simulink model "A5_model_controller"  (R2025b)
settings: Solver=VariableStepAuto  StartTime=0.0  StopTime=timeSim  FixedStep=0.00001  MaxStep=1e-3  RelTol=1e-3
undefined symbols (not defined in the file): Bf, Bk, Br, Cf, Ck, Ckappa, Cr, Cyf, Cyr, Df, Dk, Dr, eps_num, h, Izz, Jw, K_aug, K_T, Kr_T, lf, lr, m, Rw, tr, vx
libraries: simulink_extras x3, cstblocks x1
settings Model: Creator=jofr  LastModifiedBy=danilo
settings SolverCC: AlgebraicLoopSolver=TrustRegion
settings DataIOCC: LimitDataPoints=on  SaveFormat=Array  SignalLoggingSaveFormat=ModelDataLogs  ReturnWorkspaceOutputs=off
settings OptimizationCC: BlockReduction=off  BooleanDataType=off  DefaultParameterBehavior=Inlined  BufferReuse=off  LifeSpan=inf
settings DebuggingCC: SaveWithParameterizedLinksMsg=none  UnderspecifiedInitializationDetection=Classic  MergeDetectMultiDrivingBlocksExec=none  SignalResolutionControl=TryResolveAllWithWarning  MultiTaskDSMMsg=warning  MultiTaskCondExecSysMsg=none  UnconnectedInputMsg=warning  UnconnectedOutputMsg=warning  UnconnectedLineMsg=warning  InitInArrayFormatMsg=none  SFUnexpectedBacktrackingDiag=warning  SFNoUnconditionalDefaultTransitionDiag=warning  SFExecutionAtInitializationDiag=none  ArithmeticOperatorsInVariantConditions=warning
settings HardwareCC: ProdBitPerPointer=32.0  ProdBitPerSizeT=32.0  ProdBitPerPtrDiffT=32.0  ProdLargestAtomicFloat=None  ProdIntDivRoundTo=Undefined  ProdEndianess=Unspecified  ProdWordSize=32.0  ProdHWDeviceType=32-bit Generic  TargetUnknown=on
settings ModelReferenceCC: EnableRefExpFcnMdlSchedulingChecks=on  PropagateSignalLabelsOutOfModel=off
settings SFSimCC: SimUseLocalCustomCode=off  CustomCodeUndefinedFunction=UseInterfaceOnly
settings RTWCC: RTWUseLocalCustomCode=off  GPUComputeCapability=3.5  DLArmComputeVersion=19.05
settings CodeAppCC: StateflowObjectComments=on
settings GRTTargetCC: TargetLangStandard=C89/C90 (ANSI)
settings ConfigComp: CovMetricSettings=dw  CovSaveCumulativeToWorkspaceVar=on  CovSaveSingleToWorkspaceVar=on  CovExternalEMLEnable=off

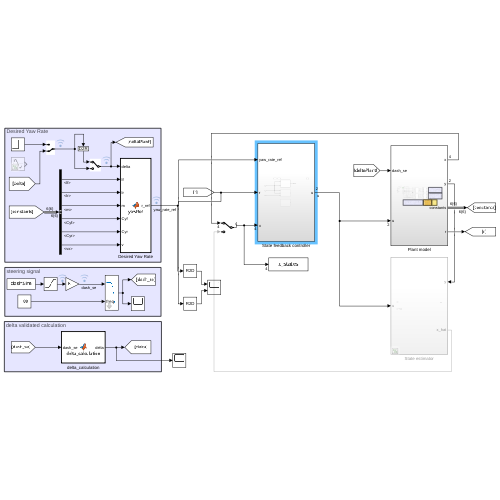
[thumbnail: Simulink's stored preview of the top-level diagram]
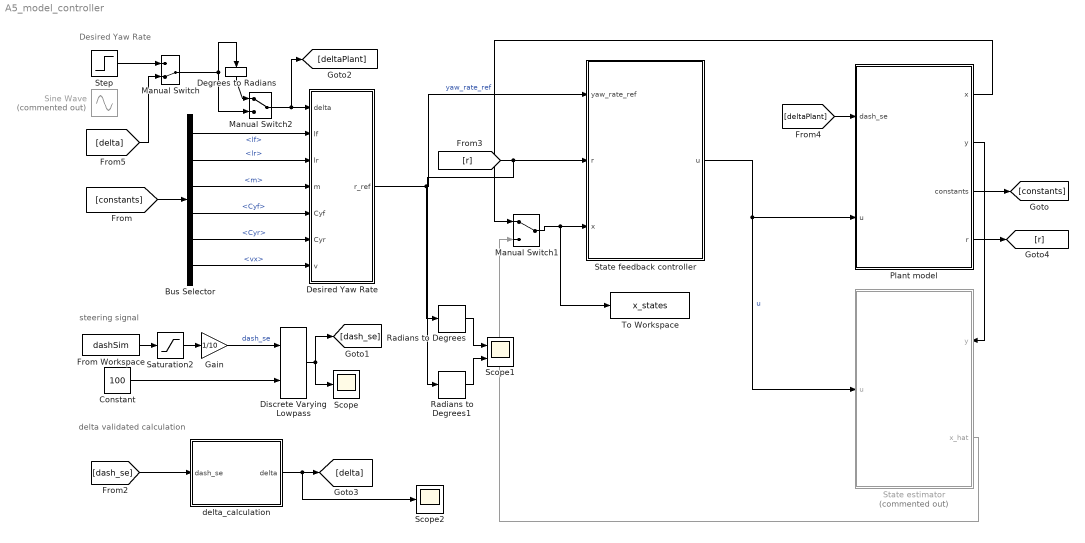
== system A5_model_controller ==
  note: delta validated calculation
  note: steering signal
  note: Desired Yaw Rate
  Bus Selector : BusSelector  OutputSignals=lf,lr,m,Cyf,Cyr,vx
  Constant : Constant  Value=100
  Degrees to Radians : simulink_extras/Transformations/Degrees to Radians
  Desired Yaw Rate : MATLAB Function  TreatAsAtomicUnit=on
  Discrete Varying Lowpass : cstblocks/Linear Parameter Varying/Discrete Varying Lowpass  N=1  w0=0  Ts=0.01
  From Workspace : FromWorkspace  VariableName=dashSim
  Gain : Gain  Gain=1/10
  Manual Switch : ManualSwitch  CurrentSetting=0
  Manual Switch1 : ManualSwitch
  Manual Switch2 : ManualSwitch
  Plant model : Subsystem
  Radians to Degrees : simulink_extras/Transformations/Radians to Degrees
  Radians to Degrees1 : simulink_extras/Transformations/Radians to Degrees
  Saturation2 : Saturate  UpperLimit=1270  LowerLimit=-1270
  Scope : Scope
      settings: ActiveDisplayYMinimum=-354.89564145632545  ActiveDisplayYMaximum=435.3727455414014  DataLoggingVariableName=ScopeData13
  Scope1 : Scope  NumInputPorts=2
      settings: ActiveDisplayYMinimum=-206.00372470004959  ActiveDisplayYMaximum=1854.0335223004467  DataLoggingVariableName=ScopeData12
  Scope2 : Scope
      settings: ActiveDisplayYMinimum=-1  ActiveDisplayYMaximum=1  DataLoggingVariableName=ScopeData18
  Sine Wave : Sin  Commented=on  Amplitude=10*(pi()/180)  Frequency=5  SampleTime=0
  State estimator : Subsystem  Commented=on
      settings: PortSchema="{\"entries\":[{\"content\":{\"sides\":[{\"content\":{\"connectorIds\":[\"In1\"]},\"type\":\"ConnectorPlacement.EquallySpacedRectSide\",\"uuid\":\"c417f3d4-912d-40bf-9a3a-53ea69fe223c\"},{\"content\":{\"connectorIds\":[\"In2\",\"Out1\"],\"side\":\"RIGHT\"},\"type\":\"ConnectorPlacement.EquallySpacedRectSide\",\"uuid\":\"4e25e672-d4ae-48e6-baf9-37985f0fdcbd\"},{\"content\":{\"connectorIds\":[],\"side\":\"TOP\"},\"type\":\"ConnectorPlacement.EquallySpacedRectSide\",\"uuid\":\"19dfc206-a33d-4b15-9300-bad270a3e9d6\"},{\"content\":{\"connectorIds\":[],\"side\":\"HIDDEN\"},\"type\":\"ConnectorPlacement.EquallySpacedRectSide\",\"uuid\":\"ab455fac-7bff-4c9f-9be5-2f044e5e011f\"}]},\"type\":\"ConnectorPlacement.EquallySpacedConnector\",\"uuid\":\"aea33454-8eab-4b9c-b4de-a2355e2c58aa\"}],\"packageUris\":[\"http://schema.mathworks.com/mf0/Connector/R2020b\"],\"version\":\"1.0\"}"
  State feedback controller : Subsystem
  Step : Step  SampleTime=0
  To Workspace : ToWorkspace  VariableName=x_states  SaveFormat=Structure With Time  SampleTime=-1
  delta_calculation : MATLAB Function  TreatAsAtomicUnit=on
  wires:
  State feedback controller/1(u) -> State estimator/1(u), Plant model/2(u)  "u"
  Plant model/2(y) -> State estimator/2(y)
  Manual Switch1/1 -> To Workspace/1, State feedback controller/3(x)
  State estimator/1(x_hat) -> Manual Switch1/2
  Plant model/1(x) -> Manual Switch1/1
  Plant model/3(constants) -> [constants]
  [constants] -> Bus Selector/1
  Bus Selector/1 -> Desired Yaw Rate/2(lf)  "<lf>"
  Bus Selector/2 -> Desired Yaw Rate/3(lr)  "<lr>"
  Bus Selector/3 -> Desired Yaw Rate/4(m)  "<m>"
  Bus Selector/4 -> Desired Yaw Rate/5(Cyf)  "<Cyf>"
  Bus Selector/5 -> Desired Yaw Rate/6(Cyr)  "<Cyr>"
  Bus Selector/6 -> Desired Yaw Rate/7(v)  "<vx>"
  From Workspace/1 -> Saturation2/1
  Saturation2/1 -> Gain/1
  Gain/1 -> Discrete Varying Lowpass/1  "dash_se"
  Discrete Varying Lowpass/1 -> [dash_se], Scope/1
  Constant/1 -> Discrete Varying Lowpass/2
  Manual Switch/1 -> Manual Switch2/2, Degrees to Radians/1
  Degrees to Radians/1 -> Manual Switch2/1
  Manual Switch2/1 -> [deltaPlant], Desired Yaw Rate/1(delta)
  Step/1 -> Manual Switch/1
  Desired Yaw Rate/1(r_ref) -> Radians to Degrees/1, State feedback controller/1(yaw_rate_ref)  "yaw_rate_ref"
  [dash_se] -> delta_calculation/1(dash_se)
  delta_calculation/1(delta) -> Scope2/1, [delta]
  Plant model/4(r) -> [r]
  [r] -> Radians to Degrees1/1, State feedback controller/2(r)
  Radians to Degrees/1 -> Scope1/1
  Radians to Degrees1/1 -> Scope1/2
  [deltaPlant] -> Plant model/1(dash_se)
  [delta] -> Manual Switch/2

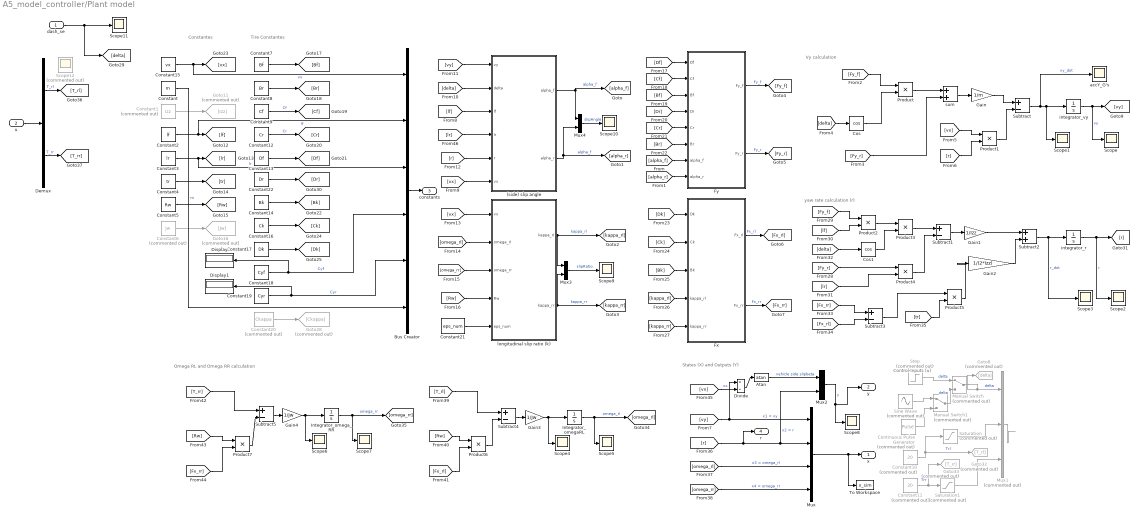
== system A5_model_controller/Plant model ==
  note: Constantes
  note: Omega RL and Omega RR calculation
  note: Control Inputs (u)
  note: States (X) and Outputs (Y)
  note: yaw rate calculation (r)
  note: Vy calculation
  note: Tire Constantes
  dash_se : Inport
  u : Inport  Port=2  PortDimensions=2
  (side) slip angle : MATLAB Function  TreatAsAtomicUnit=on
  Atan : Trigonometry  Operator=atan
  Bus Creator : BusCreator  Inputs=6
  Constant : Constant  Value=m
  Constant1 : Constant  Commented=on  Value=Izz
  Constant10 : Constant  Commented=on  Value=20
  Constant11 : Constant  Commented=on  Value=20
  Constant12 : Constant  Value=Cr
  Constant13 : Constant  Value=Df
  Constant14 : Constant  Value=Bk
  Constant15 : Constant  Value=vx
  Constant16 : Constant  Value=Ck
  Constant17 : Constant  Value=Dk
  Constant18 : Constant  Value=Cyf
  Constant19 : Constant  Value=Cyr
  Constant2 : Constant  Value=lf
  Constant20 : Constant  Commented=on  Value=Ckappa
  Constant21 : Constant  Value=eps_num
  Constant22 : Constant  Value=Dr
  Constant3 : Constant  Value=lr
  Constant4 : Constant  Value=tr
  Constant5 : Constant  Value=Rw
  Constant6 : Constant  Commented=on  Value=Jw
  Constant7 : Constant  Value=Bf
  Constant8 : Constant  Value=Br
  Constant9 : Constant  Value=Cf
  Continuous Pulse Generator : DiscretePulseGenerator  Commented=on  PulseType=Time based  Period=1  PulseWidth=50
  Cos : Trigonometry  Operator=cos
  Cos1 : Trigonometry  Operator=cos
  Demux : Demux  Outputs=2
  Display : Display
  Display1 : Display
  Divide : Product  Inputs=*/
  Fx : MATLAB Function  TreatAsAtomicUnit=on
  Fy : MATLAB Function  TreatAsAtomicUnit=on
  Gain : Gain  Gain=1/m
  Gain1 : Gain  Gain=1/Izz
  Gain2 : Gain  Gain=1/(2*Izz)
  Gain3 : Gain  Gain=1/Jw
  Gain4 : Gain  Gain=1/Jw
  Goto11 : Goto  Commented=on  GotoTag=Izz
  Goto16 : Goto  Commented=on  GotoTag=Jw
  Goto28 : Goto  Commented=on  GotoTag=Ckappa
  Goto32 : Goto  Commented=on  GotoTag=T_rl
  Goto33 : Goto  Commented=on  GotoTag=T_rr
  Goto8 : Goto  Commented=on  GotoTag=delta
  Integrator_omegaRL : Integrator  InitialCondition=vx/Rw
  Integrator_omega_RR : Integrator  InitialCondition=vx/Rw
  Manual Switch : ManualSwitch  Commented=on
  Manual Switch1 : ManualSwitch  Commented=on
  Mux : Mux
  Mux1 : Mux  Commented=on  Inputs=3
  Mux2 : Mux  Inputs=2
  Mux3 : Mux  Inputs=2
  Mux4 : Mux  Inputs=2
  Product{,1..7} (8 alike) : Product
  Saturation : Saturate  Commented=on
  Saturation1 : Saturate  Commented=on
  Scope{,1..11} (12 alike) : Scope
      Scope settings: ActiveDisplayYMinimum=-1  ActiveDisplayYMaximum=1
      Scope10 settings: ActiveDisplayYMinimum=-1  ActiveDisplayYMaximum=1  DataLoggingVariableName=ScopeData10
      Scope11 settings: DataLoggingVariableName=ScopeData14
      Scope2 settings: ActiveDisplayYMinimum=-11.738874514113046  ActiveDisplayYMaximum=1.5902174171245722  DataLoggingVariableName=ScopeData2
      Scope3 settings: DataLoggingVariableName=ScopeData3
      Scope4 settings: ActiveDisplayYMinimum=-1  ActiveDisplayYMaximum=1  DataLoggingVariableName=ScopeData4
      Scope5 settings: ActiveDisplayYMinimum=-1  ActiveDisplayYMaximum=1  DataLoggingVariableName=ScopeData5
      Scope6 settings: ActiveDisplayYMinimum=-1  ActiveDisplayYMaximum=1  DataLoggingVariableName=ScopeData6
      Scope7 settings: ActiveDisplayYMinimum=-1  ActiveDisplayYMaximum=1  DataLoggingVariableName=ScopeData7
      Scope8 settings: ActiveDisplayYMinimum=-1  ActiveDisplayYMaximum=1  DataLoggingVariableName=ScopeData8
      Scope9 settings: ActiveDisplayYMinimum=-1  ActiveDisplayYMaximum=1  DataLoggingVariableName=ScopeData9
  Scope12 : Scope  Commented=on
      settings: ActiveDisplayYMinimum=-0.01610091878561485  ActiveDisplayYMaximum=0.0017936004292760203  DataLoggingVariableName=ScopeData15
  Sine Wave : Sin  Commented=on  SampleTime=0
  Step : Step  Commented=on  SampleTime=0
  Subtract{,1,3..5} (5 alike) : Sum  Inputs=+-
  Subtract2 : Sum
  To Workspace : ToWorkspace  VariableName=x_sim  SaveFormat=Structure With Time  SampleTime=-1
  accY_G's : Scope
      settings: DataLoggingVariableName=ScopeData11
  integrator_r : Integrator
  integrator_vy : Integrator
  "longitudinal slip ratio (k) " : MATLAB Function  TreatAsAtomicUnit=on
  sum : Sum
  x : Outport
  y : Outport  Port=2
  constants : Outport  Port=3
  r : Outport  Port=4
  wires:
  [vy] -> Divide/1, Mux/1  "x1 = vy"
  [r] -> r/1, Mux/2, Mux2/2  "x2 = r"
  Constant10/1 -> Saturation/1, Goto32/1  "Trl"
  Constant11/1 -> Goto33/1, Saturation1/1  "Trr"
  (side) slip angle/1(alpha_f) -> [alpha_f], Mux4/1  "alpha_f"
  (side) slip angle/2(alpha_r) -> Mux4/2, [alpha_r]  "alpha_f"
  "longitudinal slip ratio (k) "/1(kappa_rl) -> [kappa_rl], Mux3/1  "kappa_rl"
  "longitudinal slip ratio (k) "/2(kappa_rr) -> [kappa_rr], Mux3/2  "kappa_rr"
  Fy/1(Fy_f) -> [Fy_f]  "Fy_f"
  Fy/2(Fy_r) -> [Fy_r]  "Fy_r"
  Fx/1(Fx_rl) -> [Fx_rl]  "Fx_rl"
  Fx/2(Fx_rr) -> [Fx_rr]  "Fx_rr"
  [alpha_f] -> Fy/7(alpha_f)
  [alpha_r] -> Fy/8(alpha_r)
  [delta] -> Cos/1
  [Fy_f] -> Product/1
  Cos/1 -> Product/2
  Product/1 -> sum/1
  [Fy_r] -> sum/2
  sum/1 -> Gain/1
  Gain/1 -> Subtract/1
  [vx] -> Product1/1
  [r] -> Product1/2
  Product1/1 -> Subtract/2
  Subtract/1 -> accY_G's/1, Scope1/1, integrator_vy/1  "vy_dot"
  integrator_vy/1 -> Scope/1, [vy]  "vy"
  Constant1/1 -> Goto11/1
  Constant2/1 -> [lf], Bus Creator/2  "lf"
  Constant3/1 -> [lr], Bus Creator/3  "lr"
  Constant4/1 -> [tr]
  Constant5/1 -> [Rw]
  Constant6/1 -> Goto16/1
  Constant7/1 -> [Bf]
  Constant8/1 -> [Br]
  Constant9/1 -> [Cf]  "Cf"
  Constant12/1 -> [Cr]  "Cr"
  Constant13/1 -> [Df]
  Constant14/1 -> [Bk]
  Constant15/1 -> Bus Creator/1, [vx]  "vx"
  Constant16/1 -> [Ck]
  Constant17/1 -> [Dk]
  Constant18/1 -> Display/1, Bus Creator/4  "Cyf"
  Constant19/1 -> Display1/1, Bus Creator/5  "Cyr"
  Constant20/1 -> Goto28/1
  [vx] -> (side) slip angle/6(vx)
  [vy] -> (side) slip angle/1(vy)
  [delta] -> (side) slip angle/2(delta)
  [lf] -> (side) slip angle/3(lf)
  [r] -> (side) slip angle/5(r)
  [vx] -> "longitudinal slip ratio (k) "/1(vx)
  [omega_rl] -> "longitudinal slip ratio (k) "/2(omega_rl)
  [Rw] -> "longitudinal slip ratio (k) "/4(Rw)
  [omega_rr] -> "longitudinal slip ratio (k) "/3(omega_rr)
  [Df] -> Fy/1(Df)
  [Cf] -> Fy/2(Cf)
  [Bf] -> Fy/3(Bf)
  [Dr] -> Fy/4(Dr)
  [Cr] -> Fy/5(Cr)
  [Br] -> Fy/6(Br)
  Constant22/1 -> [Dr]
  Saturation/1 -> Mux1/2
  Saturation1/1 -> Mux1/3
  [Dk] -> Fx/1(Dk)
  [Ck] -> Fx/2(Ck)
  [Bk] -> Fx/3(Bk)
  [kappa_rl] -> Fx/4(kappa_rl)
  [kappa_rr] -> Fx/5(kappa_rr)
  [delta] -> Cos1/1
  [Fy_f] -> Product2/1
  [lf] -> Product2/2
  Cos1/1 -> Product3/2
  Product2/1 -> Product3/1
  [Fy_r] -> Product4/1
  [lr] -> Product4/2
  Product4/1 -> Subtract1/2
  Product3/1 -> Subtract1/1
  Subtract1/1 -> Gain1/1
  [Fx_rr] -> Subtract3/1
  [Fx_rl] -> Subtract3/2
  Subtract3/1 -> Product5/1
  [tr] -> Product5/2
  Product5/1 -> Gain2/1
  Gain2/1 -> Subtract2/2
  Subtract2/1 -> Scope3/1, integrator_r/1  "r_dot"
  [Rw] -> Product6/1
  [Fx_rl] -> Product6/2
  Product6/1 -> Subtract4/2
  [T_rl] -> Subtract4/1
  Subtract4/1 -> Gain3/1
  Gain3/1 -> Scope4/1, Integrator_omegaRL/1
  Integrator_omegaRL/1 -> Scope5/1, [omega_rl]  "omega_rl"
  Integrator_omega_RR/1 -> [omega_rr], Scope7/1  "omega_rr"
  Gain4/1 -> Integrator_omega_RR/1, Scope6/1
  Subtract5/1 -> Gain4/1
  [T_rr] -> Subtract5/1
  Product7/1 -> Subtract5/2
  [Fx_rr] -> Product7/2
  [Rw] -> Product7/1
  Mux2/1 -> Scope8/1, y/1  "y"
  Atan/1 -> Mux2/1  "vehicle side slipbeta"
  Divide/1 -> Atan/1
  [vx] -> Divide/2  "vx"
  Constant/1 -> Bus Creator/6  "m"
  [lr] -> (side) slip angle/4(lr)
  Mux3/1 -> Scope9/1  "slipRatio"
  Mux4/1 -> Scope10/1  "slipAngle"
  Manual Switch/1 -> Goto8/1, Mux1/1  "delta"
  Step/1 -> Manual Switch/1  "delta"
  Continuous Pulse Generator/1 -> Manual Switch1/2
  Manual Switch1/1 -> Manual Switch/2  "delta"
  Sine Wave/1 -> Manual Switch1/1
  Mux1/1 -> ?
  u/1 -> Demux/1
  Constant21/1 -> "longitudinal slip ratio (k) "/5(eps_num)
  Bus Creator/1 -> constants/1
  Mux/1 -> To Workspace/1, x/1
  Gain1/1 -> Subtract2/1
  integrator_r/1 -> Scope2/1, [r]  "r"
  [omega_rl] -> Mux/3  "x3 = omega_rl"
  [omega_rr] -> Mux/4  "x4 = omega_rr"
  dash_se/1 -> [delta], Scope11/1
  Demux/1 -> [T_rl]  "T_rl"
  Demux/2 -> [T_rr]  "T_rr"

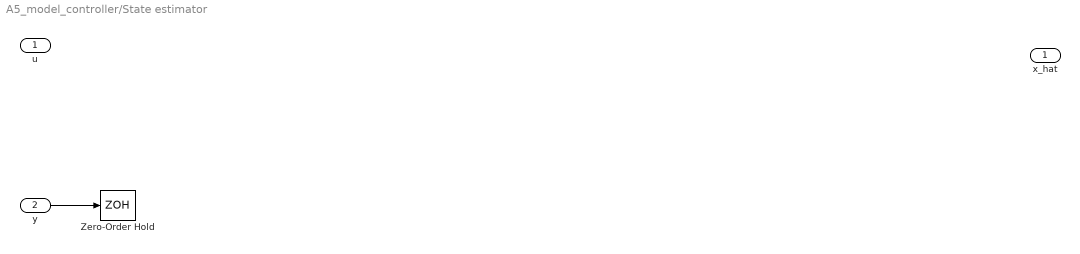
== system A5_model_controller/State estimator ==
  u : Inport
  y : Inport  Port=2
  Zero-Order Hold : ZeroOrderHold  SampleTime=h
  x_hat : Outport
  wires:
  y/1 -> Zero-Order Hold/1

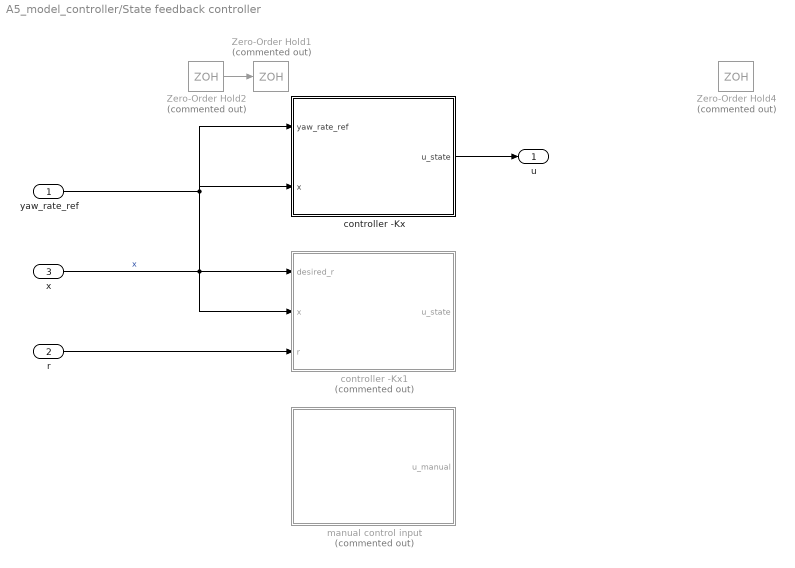
== system A5_model_controller/State feedback controller ==
  yaw_rate_ref : Inport
  r : Inport  Port=2
  x : Inport  Port=3
  Zero-Order Hold1 : ZeroOrderHold  Commented=on  SampleTime=h
  Zero-Order Hold2 : ZeroOrderHold  Commented=on  SampleTime=h
  Zero-Order Hold4 : ZeroOrderHold  Commented=on  SampleTime=-1
  controller -Kx : Subsystem
  controller -Kx1 : Subsystem  Commented=on
  manual control input : Subsystem  Commented=on
  u : Outport  PortDimensions=2
  wires:
  Zero-Order Hold2/1 -> Zero-Order Hold1/1
  yaw_rate_ref/1 -> controller -Kx1/1(desired_r), controller -Kx/1(yaw_rate_ref)
  x/1 -> controller -Kx/2(x), controller -Kx1/2(x)  "x"
  r/1 -> controller -Kx1/3(r)
  controller -Kx/1(u_state) -> u/1

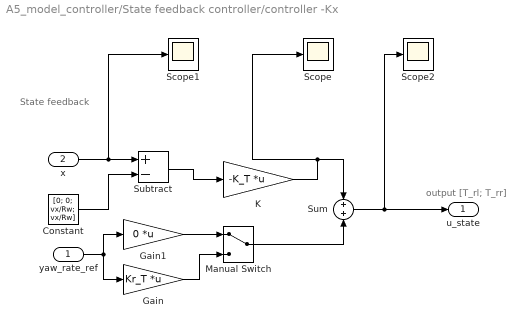
== system A5_model_controller/State feedback controller/controller -Kx ==
  note: output [T_rl; T_rr]
  note: State feedback
  yaw_rate_ref : Inport
  x : Inport  Port=2  PortDimensions=4
  Constant : Constant  Value=[0; 0; vx/Rw; vx/Rw]  VectorParams1D=off
  Gain : Gain  Gain=Kr_T  Multiplication=Matrix(K*u)
  Gain1 : Gain  Gain=0  Multiplication=Matrix(K*u)
  K : Gain  Gain=-K_T  Multiplication=Matrix(K*u)
  Manual Switch : ManualSwitch
  Scope : Scope
      settings: ActiveDisplayYMinimum=-0.0010140194157633876  ActiveDisplayYMaximum=0.0010146249929807261  DataLoggingVariableName=ScopeData16
  Scope1 : Scope
      settings: ActiveDisplayYMinimum=-6.7509721632618485  ActiveDisplayYMaximum=49.483096533791262  DataLoggingVariableName=ScopeData17
  Scope2 : Scope
      settings: ActiveDisplayYMinimum=-0.41126063504540261  ActiveDisplayYMaximum=0.41126063504546317  DataLoggingVariableName=ScopeData19
  Subtract : Sum  Inputs=+-
  Sum : Sum
  u_state : Outport  PortDimensions=2
  wires:
  x/1 -> Subtract/1, Scope1/1
  K/1 -> Scope/1, Sum/1
  Sum/1 -> Scope2/1, u_state/1
  Gain/1 -> Manual Switch/2
  yaw_rate_ref/1 -> Gain/1, Gain1/1
  Manual Switch/1 -> Sum/2
  Gain1/1 -> Manual Switch/1
  Subtract/1 -> K/1
  Constant/1 -> Subtract/2

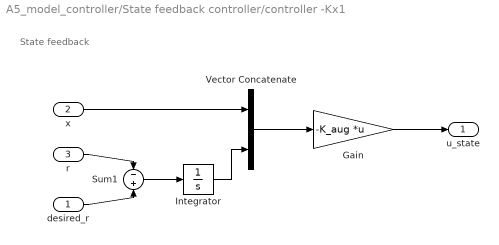
== system A5_model_controller/State feedback controller/controller -Kx1 ==
  note: State feedback
  desired_r : Inport
  x : Inport  Port=2  PortDimensions=4
  r : Inport  Port=3
  Gain : Gain  Gain=-K_aug  Multiplication=Matrix(K*u)
  Integrator : Integrator
  Sum1 : Sum  Inputs=-+
  Vector Concatenate : Concatenate
  u_state : Outport
  wires:
  desired_r/1 -> Sum1/2
  x/1 -> Vector Concatenate/1
  r/1 -> Sum1/1
  Sum1/1 -> Integrator/1
  Vector Concatenate/1 -> Gain/1
  Integrator/1 -> Vector Concatenate/2
  Gain/1 -> u_state/1

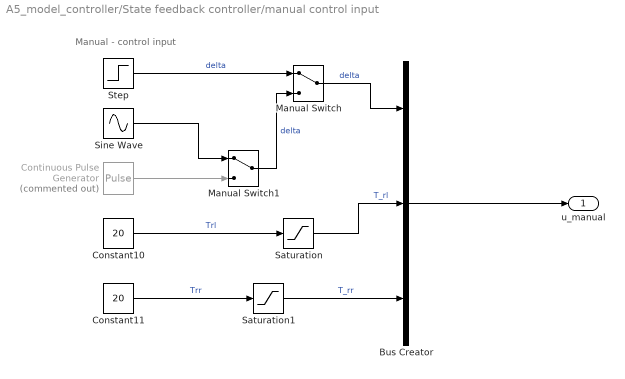
== system A5_model_controller/State feedback controller/manual control input ==
  note: Manual - control input
  Bus Creator : BusCreator  Inputs=3
  Constant10 : Constant  Value=20
  Constant11 : Constant  Value=20
  Continuous Pulse Generator : DiscretePulseGenerator  Commented=on  PulseType=Time based  Period=1  PulseWidth=50
  Manual Switch : ManualSwitch
  Manual Switch1 : ManualSwitch
  Saturation : Saturate
  Saturation1 : Saturate
  Sine Wave : Sin  SampleTime=0
  Step : Step  SampleTime=0
  u_manual : Outport
  wires:
  Sine Wave/1 -> Manual Switch1/1
  Manual Switch/1 -> Bus Creator/1  "delta"
  Constant11/1 -> Saturation1/1  "Trr"
  Continuous Pulse Generator/1 -> Manual Switch1/2
  Manual Switch1/1 -> Manual Switch/2  "delta"
  Saturation1/1 -> Bus Creator/3  "T_rr"
  Saturation/1 -> Bus Creator/2  "T_rl"
  Constant10/1 -> Saturation/1  "Trl"
  Bus Creator/1 -> u_manual/1
  Step/1 -> Manual Switch/1  "delta"

== matlab function A5_model_controller/Plant model/longitudinal slip ratio (k)  ==
  data: vx input; kappa_rl output; omega_rl input; omega_rr input; Rw input; kappa_rr output; eps_num input
function [kappa_rl,kappa_rr] = slipRatio(vx,omega_rl,omega_rr,Rw,eps_num)
kappa_rl = (Rw*omega_rl - vx)/(vx + eps_num);
kappa_rr = (Rw*omega_rr - vx)/(vx + eps_num);
end

== matlab function A5_model_controller/Plant model/(side) slip angle ==
  data: vy input; alpha_f output; delta input; lf input; lr input; r input; vx input; alpha_r output
 function [alpha_f,alpha_r] = slipAngles(vy,delta,lf,lr,r,vx)
alpha_f = atan( (vy + lf*r)/vx ) - delta;
alpha_r = atan( (vy - lr*r)/vx );
end

== matlab function A5_model_controller/Plant model/Fy ==
  data: Df input; Cf input; Fy_f output; Bf input; Dr input; Cr input; Br input; alpha_f input; Fy_r output; alpha_r input
function [Fy_f, Fy_r] = FyTire(Df,Cf,Bf,Dr,Cr,Br,alpha_f,alpha_r)
%#codegen
Fy_f = -2.*Df .* sin( Cf .* atan( Bf .* alpha_f ) );
Fy_r = -2.*Dr .* sin( Cr .* atan( Br .* alpha_r ) );
end

== matlab function A5_model_controller/Plant model/Fx ==
  data: Dk input; Ck input; Fx_rl output; Bk input; kappa_rl input; kappa_rr input; Fx_rr output
function [Fx_rl,Fx_rr] = FxTire(Dk,Ck,Bk,kappa_rl,kappa_rr)
Fx_rl =  Dk .* sin( Ck .* atan( Bk .* kappa_rl ) );
Fx_rr =  Dk .* sin( Ck .* atan( Bk .* kappa_rr ) );
end

== matlab function A5_model_controller/Desired Yaw Rate ==
  data: delta input; lf input; lr input; m input; Cyf input; Cyr input; r_ref output; v input
function r_ref = yawRef(delta, lf, lr, m,Cyf, Cyr, v)
g = 9.81; 
L = lf + lr;
Kus = (m/L)*(lr/Cyr - lf/Cyf);     % >0 => understeer
r_ref = delta * ( v / ( L + (Kus/g)*v^2 ) );

== matlab function A5_model_controller/delta_calculation ==
  data: dash_se input; delta output
function delta = delta_calculation(dash_se)
dash = dash_se;
if dash > 0
    delta = (1)*(5*power(10,-6) * power(dash,2) + 0.0039*dash - 0.0002);
else
    delta = (1)*(3*power(10,-6) * power(dash,2) + 0.0039*dash - 0.0027);
end
